simulink model "LCK_old"  (R2018b)
settings: Solver=FixedStepDiscrete  StartTime=0.0  StopTime=inf  FixedStep=0.005  RelTol=1e-3
PostLoadFcn:
  | if any(exist('dsrtsu_mdlpostloadfcn', 'file') ~= 0), dsrtsu_mdlpostloadfcn('Execute', bdroot); end
values from neighbouring files (symbols this model uses):
  C_DEG2RAD = 0.0175    [LCK_Macro.sldd]
  C_KPH2MPS = 0.2778    [LCK_Macro.sldd]
  C_NEARZERO = 0.0001    [LCK_Macro.sldd]
  C_ONE = 1.0    [LCK_Macro.sldd]
  C_RAD2DEG = 57.2958    [LCK_Macro.sldd]
  C_ZERO = 0.0    [LCK_Macro.sldd]
  k_accel_pedal_pos_per_speed_x : value not decoded    [LCK_LogicPara.sldd]
  k_accel_pedal_pos_per_speed_z : value not decoded    [LCK_LogicPara.sldd]
  k_brake_suprress_hold = 1000.0    [LCK_LogicPara.sldd]
  k_driver_appl_torque_filt = 50.0    [LCK_LogicPara.sldd]
  k_driver_suppression_hold_time = 3000.0    [LCK_LogicPara.sldd]
  k_hands_on_wheel_hold_msec = 500.0    [LCK_LogicPara.sldd]
  k_hands_on_wheel_torque_hi = 0.2    [LCK_LogicPara.sldd]
  k_hands_on_wheel_torque_lo = 0.15    [LCK_LogicPara.sldd]
  k_handsoff_delay_cycles = 50.0    [LCK_LogicPara.sldd]
  k_handsoff_torq_Lo_CR = 0.3    [LCK_LogicPara.sldd]
  k_handson_delay_cycles = 5.0    [LCK_LogicPara.sldd]
  k_HighAccel_suppress_hold = 3000.0    [LCK_LogicPara.sldd]
  k_HLR_suprress_hold = 3000.0    [LCK_LogicPara.sldd]
  k_hs_StrAng_CR_threshold_z : value not decoded    [LCK_LogicPara.sldd]
  k_LC_Exit_Switch = 0.0    [LCK_LogicPara.sldd]
  k_LCG_Configured = 1.0    [LCK_LogicPara.sldd]
  k_LCK_A0_Rdy2Act_UseConst = 0.0    [LCK_LogicPara.sldd]
  k_LCK_A0Fac_ActSta : value not decoded    [LCK_CtrlPara.sldd]
  k_LCK_A0Fac_DrvStm : value not decoded    [LCK_CtrlPara.sldd]
  k_LCK_A0Shift_LftCurv : value not decoded    [LCK_CtrlPara.sldd]
  k_LCK_A0Shift_RgtCurv : value not decoded    [LCK_CtrlPara.sldd]
  k_LCK_A0Shift_StraLan = 0.0    [LCK_CtrlPara.sldd]
  k_LCK_A0ShiftFac_Dy_LftCurv : value not decoded    [LCK_CtrlPara.sldd]
  k_LCK_A0ShiftFac_Dy_RgtCurv : value not decoded    [LCK_CtrlPara.sldd]
  k_LCK_A0ShiftFac_Vspd : value not decoded    [LCK_CtrlPara.sldd]
  k_LCK_accel_inhibit_thold = 35.0    [LCK_LogicPara.sldd]
  k_LCK_Active2Ready_Mask = 255.0    [LCK_LogicPara.sldd]
  k_LCK_CvatRateBks : value not decoded    [LCK_CtrlPara.sldd]
  k_LCK_CvatrBks : value not decoded    [LCK_CtrlPara.sldd]
  k_LCK_DFac_Dy : value not decoded    [LCK_CtrlPara.sldd]
  k_LCK_DFac_Dy_Curv : value not decoded    [LCK_CtrlPara.sldd]
  k_LCK_DFac_HaCurCen : value not decoded    [LCK_CtrlPara.sldd]
  k_LCK_DFac_HaCurSid : value not decoded    [LCK_CtrlPara.sldd]
  k_LCK_DFac_HadCurCen : value not decoded    [LCK_CtrlPara.sldd]
  k_LCK_DFac_HadCurSid : value not decoded    [LCK_CtrlPara.sldd]
  k_LCK_DFac_HadStrCen : value not decoded    [LCK_CtrlPara.sldd]
  k_LCK_DFac_HadStrSid : value not decoded    [LCK_CtrlPara.sldd]
  k_LCK_DFac_HaStrCen : value not decoded    [LCK_CtrlPara.sldd]
  k_LCK_DFac_HaStrSid : value not decoded    [LCK_CtrlPara.sldd]
  k_LCK_DFac_Rad : value not decoded    [LCK_CtrlPara.sldd]
  k_LCK_DFac_SA_CurCen : value not decoded    [LCK_CtrlPara.sldd]
  k_LCK_DFac_SA_CurSid : value not decoded    [LCK_CtrlPara.sldd]
  k_LCK_DFac_SA_StrCen : value not decoded    [LCK_CtrlPara.sldd]
  k_LCK_DFac_SA_StrSid : value not decoded    [LCK_CtrlPara.sldd]
  k_LCK_DFac_SS_CurCen : value not decoded    [LCK_CtrlPara.sldd]
  k_LCK_DFac_SS_CurSid : value not decoded    [LCK_CtrlPara.sldd]
  k_LCK_DFac_SS_StrCen : value not decoded    [LCK_CtrlPara.sldd]
  k_LCK_DFac_SS_StrSid : value not decoded    [LCK_CtrlPara.sldd]
  k_LCK_DFac_Vspd : value not decoded    [LCK_CtrlPara.sldd]
  k_LCK_DlyTm_DrvStim = 0.2    [LCK_CtrlPara.sldd]
  k_LCK_DTermMax = 2.0    [LCK_CtrlPara.sldd]
  k_LCK_DyBks_Curv : value not decoded    [LCK_CtrlPara.sldd]
  k_LCK_Enable_POOnly = 1.0    [LCK_LogicPara.sldd]
  k_LCK_Entry_DistBuffer = 0.1    [LCK_LogicPara.sldd]
  k_LCK_Fac_Vspd2RngThr_FalRec = 0.23    [LCK_CtrlPara.sldd]
  k_LCK_Ffw_CvatSwh = 0.0    [LCK_CtrlPara.sldd]
  k_LCK_Ffw_DyBks : value not decoded    [LCK_CtrlPara.sldd]
  k_LCK_Ffw_TimCon_CmdFlt = 0.0    [LCK_CtrlPara.sldd]
  k_LCK_FfwDeltaFac_Rad_Lft : value not decoded    [LCK_CtrlPara.sldd]
  k_LCK_FfwDeltaFac_Rad_Rgt : value not decoded    [LCK_CtrlPara.sldd]
  k_LCK_FfwDeltaFac_Vspd : value not decoded    [LCK_CtrlPara.sldd]
  k_LCK_FfwFac_CvatRate_Lft : value not decoded    [LCK_CtrlPara.sldd]
  k_LCK_FfwFac_CvatRate_Rgt : value not decoded    [LCK_CtrlPara.sldd]
  k_LCK_FfwFac_Dy : value not decoded    [LCK_CtrlPara.sldd]
  k_LCK_FfwFac_Rad_Lft : value not decoded    [LCK_CtrlPara.sldd]
  k_LCK_FfwFac_Rad_Rgt : value not decoded    [LCK_CtrlPara.sldd]
  k_LCK_FfwFac_Vspd : value not decoded    [LCK_CtrlPara.sldd]
  k_LCK_FfwTorq_Cvat : value not decoded    [LCK_CtrlPara.sldd]
  k_LCK_HAFac_ActSta : value not decoded    [LCK_CtrlPara.sldd]
  k_LCK_HAFac_DrvStm : value not decoded    [LCK_CtrlPara.sldd]
  k_LCK_HaloTime = 2000.0    [LCK_LogicPara.sldd]
  k_LCK_HaloTime_Switch = 0.0    [LCK_LogicPara.sldd]
  k_LCK_HARFac_ActSta : value not decoded    [LCK_CtrlPara.sldd]
  k_LCK_HARFac_DrvStm : value not decoded    [LCK_CtrlPara.sldd]
  k_LCK_Hed_DyBks : value not decoded    [LCK_CtrlPara.sldd]
  k_LCK_HedAngDiffX : value not decoded    [LCK_CtrlPara.sldd]
  k_LCK_HedAngRateDiffX : value not decoded    [LCK_CtrlPara.sldd]
  k_LCK_HndsOnWhel_DlyTm_Idl2Rdy = 0.0    [LCK_LogicPara.sldd]
  k_LCK_host_veh_width = 1.86    [LCK_LogicPara.sldd]
  k_LCK_Idle2Ready_Mask = 239.0    [LCK_LogicPara.sldd]
  k_LCK_Junc_SusTime = 1.0    [LCK_LogicPara.sldd]
  k_LCK_KpKdDecSlopeLmt = 10.0    [LCK_CtrlPara.sldd]
  k_LCK_KpKdIncSlopeLmt = 5.0    [LCK_CtrlPara.sldd]
  k_LCK_Lat_Ctrl_DFac_Lft = 1.0    [LCK_CtrlPara.sldd]
  k_LCK_Lat_Ctrl_DFac_Rgt = 1.05    [LCK_CtrlPara.sldd]
  k_LCK_Lat_Ctrl_Kd = 0.8    [LCK_CtrlPara.sldd]
  k_LCK_Lat_Ctrl_Ki = 0.5    [LCK_CtrlPara.sldd]
  k_LCK_Lat_Ctrl_Kp = 0.7    [LCK_CtrlPara.sldd]
  k_LCK_Lat_Ctrl_Kp_NearGain = 0.7    [LCK_CtrlPara.sldd]
  k_LCK_Lat_Ctrl_PFac_Lft = 1.0    [LCK_CtrlPara.sldd]
  k_LCK_Lat_Ctrl_PFac_Rgt = 1.05    [LCK_CtrlPara.sldd]
  k_LCK_Lat_Ctrl_TimCon_CmdFlt = 5.0    [LCK_CtrlPara.sldd]
  k_LCK_Lat_DFac_Rad : value not decoded    [LCK_CtrlPara.sldd]
  k_LCK_Lat_DFac_SS_Cur : value not decoded    [LCK_CtrlPara.sldd]
  k_LCK_Lat_DFac_SS_Str : value not decoded    [LCK_CtrlPara.sldd]
  k_LCK_Lat_DFac_Vspd : value not decoded    [LCK_CtrlPara.sldd]
  k_LCK_Lat_DyBks : value not decoded    [LCK_CtrlPara.sldd]
  k_LCK_Lat_IFac_Rad : value not decoded    [LCK_CtrlPara.sldd]
  k_LCK_Lat_IFac_Vspd : value not decoded    [LCK_CtrlPara.sldd]
  k_LCK_Lat_ILmtFac_Dy_CurvLan : value not decoded    [LCK_CtrlPara.sldd]
  k_LCK_Lat_ILmtFac_Dy_StraLan : value not decoded    [LCK_CtrlPara.sldd]
  k_LCK_Lat_ILmtFac_Rad : value not decoded    [LCK_CtrlPara.sldd]
  k_LCK_Lat_ILmtFac_Rad_NearGain = 1.0    [LCK_CtrlPara.sldd]
  k_LCK_Lat_ILmtFac_Vspd_CurvLan : value not decoded    [LCK_CtrlPara.sldd]
  k_LCK_Lat_ILmtFac_Vspd_StraLan : value not decoded    [LCK_CtrlPara.sldd]
  k_LCK_Lat_ITermLmt_Dy = 1.0    [LCK_CtrlPara.sldd]
  k_LCK_Lat_KpKdDecSlopeLmt = 10.0    [LCK_CtrlPara.sldd]
  k_LCK_Lat_KpKdIncSlopeLmt = 10.0    [LCK_CtrlPara.sldd]
  k_LCK_Lat_PFac_Dy_InnLftCur : value not decoded    [LCK_CtrlPara.sldd]
  k_LCK_Lat_PFac_Dy_InnRgtCur : value not decoded    [LCK_CtrlPara.sldd]
  k_LCK_Lat_PFac_Dy_OutLftCur : value not decoded    [LCK_CtrlPara.sldd]
  k_LCK_Lat_PFac_Dy_OutRgtCur : value not decoded    [LCK_CtrlPara.sldd]
  k_LCK_Lat_PFac_Dy_Str : value not decoded    [LCK_CtrlPara.sldd]
  k_LCK_Lat_PFac_Rad : value not decoded    [LCK_CtrlPara.sldd]
  ... (+158 more)
undefined symbols (not defined in the file or in its folder): k_LCK_CurvBks, K_LCK_SPA0A1A2_LMRngCmp_y
libraries: LateralControl_fcns_lib x58, simulink x22
(part 30 of 45)

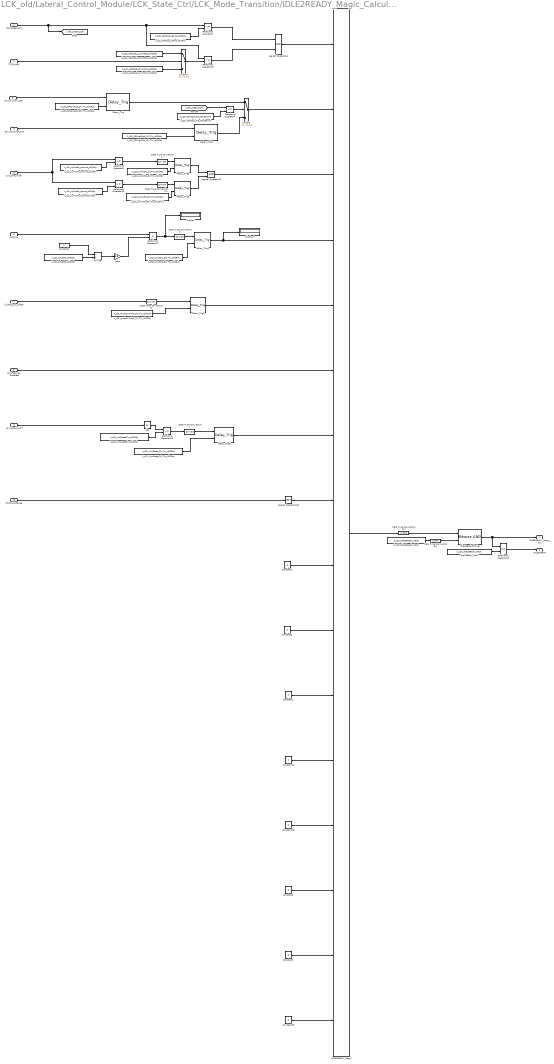
== system LCK_old/Lateral_Control_Module/LCK_State_Ctrl/LCK_Mode_Transition/IDLE2READY_Magic_Calculation ==
  Veh_Speed_kph : Inport
  TJA_Switch : Inport  Port=2
  SP_valid_low_spd : Inport  Port=3
  SP_valid_high_spd : Inport  Port=4
  curr_lane_width : Inport  Port=5
  SPP_A2 : Inport  Port=6
  f_hands_on_wheel : Inport  Port=7
  LCK_Feature_Enabled : Inport  Port=8
  yaw_deg_iso_filt : Inport  Port=9
  Short_LM_Range : Inport  Port=10
  Abs : Abs  Tag={'output',{'type','Float32'},'date',737293.69073196757}  Description=_GWMAB30P4.LCK.000_115_
  Constant1 : Constant  Tag={'output',{'class','ESR_VC/CONST','type','UInt16'},'date',737194.71790592594}  Description=_GWMAB30P2.LCK.000_1070_  Value=0
  Constant11 : Constant  Tag={'output',{'type','Int32'},'date',737237.63745895831}  Description=_GWMAB30P3.LCK.000_18_  Value=0
  Constant15 : Constant  Tag={'output',{'type','Int32'},'date',737504.55055067129}  Description=_GWMAB30P3.LCK.000_21_  Value=0
  Constant16 : Constant  Tag={'output',{'type','Int32'},'date',737237.63745961804}  Description=_GWMAB30P3.LCK.000_22_  Value=0
  Constant2 : Constant  Tag={'output',{'class','ESR_VC/CONST','type','UInt16'},'date',737194.71790592594}  Description=_GWMAB30P2.LCK.000_1070_  Value=0
  Constant3 : Constant  Tag={'output',{'class','ESR_VC/CONST','type','UInt16'},'date',737504.5503860648}  Description=_GWMAB30P2.LCK.000_1079_  Value=0
  Constant4 : Constant  Tag={'output',{'type','Int32'},'date',737296.81489093753}  Description=_GWMAB30P2.LCK.000_1072_
  Constant5 : Constant  Tag={'output',{'class','ESR_VC/CONST','type','UInt16'},'date',737194.71790592594}  Description=_GWMAB30P2.LCK.000_1070_  Value=0
  Constant9 : Constant  Tag={'output',{'class','ESR_VC/CONST','type','UInt16'},'date',737194.71813111112}  Description=_GWMAB30P2.LCK.000_1085_  Value=0
  Data Type Conversion1 : DataTypeConversion  Description=_GWMAB30P4.LCK.000_121_
  Data Type Conversion11 : DataTypeConversion  Description=_GWMAB30P4.LCK.000_122_
  Data Type Conversion12 : DataTypeConversion  Description=_GWMAB30P4.LCK.000_123_  OutDataTypeStr=uint16
  Data Type Conversion21 : DataTypeConversion  Description=_GWMAB30P4.LCK.000_132_
  Data Type Conversion3 : DataTypeConversion  Description=_GWMAB30P4.LCK.000_141_
  Data Type Conversion4 : DataTypeConversion  Description=_GWMAB30P4.LCK.000_146_
  Data Type Conversion93 : DataTypeConversion  OutDataTypeStr=uint16
  Delay_Trig{,1..6} (7 alike) : LateralControl_fcns_lib/Delay_Trig  SystemSampleTime=-1
  Display : Display
  Display1 : Display
  Divide : Product  Inputs=*/
  Gain : Gain  Gain=0.5
  IDLE2READY_Magic : LateralControl_fcns_lib/Bit_To_Integer_16  SystemSampleTime=-1
  "Idle2ReadyBitwise " : simulink/Logic and Bit Operations/Bitwise Operator  logicop=AND  UseBitMask=off  NumInputPorts=2  BitMask=k_LCK_Ready2Idle_Mask  BitMaskRealWorld=Stored Integer
  Idle2Ready_Mask : Constant  Value=k_LCK_Idle2Ready_Mask  SampleTime=-1
  Logical Operator13 : Logic  Tag={'date',737184.60397620371}  Description=_GWMAB30P2.LCK.000_1095_  AllPortsSameDT=off  OutDataTypeStr=boolean
  Logical Operator160 : Logic  Operator=NOT  AllPortsSameDT=off  OutDataTypeStr=boolean
  Logical Operator44 : Logic  Tag={'date',737184.60398003471}  Description=_GWMAB30P2.LCK.000_1126_  AllPortsSameDT=off  OutDataTypeStr=boolean
  Relational Operator10 : RelationalOperator  Tag={'date',737184.60398142366}  Description=_GWMAB30P2.LCK.000_1137_  Operator=<=  OutDataTypeStr=boolean  RndMeth=Nearest
  Relational Operator11 : RelationalOperator  Tag={'date',737184.60398153937}  Description=_GWMAB30P2.LCK.000_1138_  Operator=<  OutDataTypeStr=boolean  RndMeth=Nearest
  Relational Operator15 : RelationalOperator  Tag={'date',737184.60398204857}  Description=_GWMAB30P2.LCK.000_1142_  OutDataTypeStr=boolean  RndMeth=Nearest
  Relational Operator2 : RelationalOperator  Tag={'date',737184.60398265044}  Description=_GWMAB30P2.LCK.000_1147_  Operator=<=  OutDataTypeStr=boolean  RndMeth=Nearest
  Relational Operator29 : RelationalOperator  Tag={'date',737292.69766562502}  Description=_GWMAB30P4.LCK.000_184_  Operator=<=  OutDataTypeStr=boolean  RndMeth=Nearest
  Relational Operator4 : RelationalOperator  Tag={'date',737184.60398497689}  Description=_GWMAB30P2.LCK.000_1166_  Operator=<=  OutDataTypeStr=boolean  RndMeth=Nearest
  Relational Operator9 : RelationalOperator  Tag={'date',737184.6039873379}  Description=_GWMAB30P2.LCK.000_1185_  OutDataTypeStr=boolean  RndMeth=Nearest
  Relational_Operator10 : RelationalOperator  Tag={'date',737184.60398758098}  Description=_GWMAB30P2.LCK.000_1187_  Operator===  OutDataTypeStr=boolean  RndMeth=Nearest
  Switch3 : Switch  Tag={'output',{'inheritscaling',1},'threshold',{'type','Int32','scalar',1},'date',737534.68149979168}  Description=_GWMAB30P2.LCK.000_1193_  Threshold=0.5
  Switch77 : Switch  Tag={'output',{'type','UInt16'},'threshold',{'type','Int32'},'date',737243.53815450228}  Description=_GWMAB30P3.LCK.000_111_  Threshold=0.5
  k_LCK_HndsOnWhel_DlyTm_Idl2Rdy : Constant  Tag={'output',{'name','$P','class','EXTERN_CAL','type','UInt8'},'date',737246.8645407639}  Description=_GWMAB30P2.LCK.000_1235_  Value=k_LCK_HndsOnWhel_DlyTm_Idl2Rdy
  k_LCK_Idle2Ready_Mask : Constant  Value=k_LCK_Idle2Ready_Mask
  k_LCK_LM_ROC_DlyTm_Idl2Rdy : Constant  Tag={'output',{'name','$P','class','EXTERN_CAL','type','UInt8'},'date',737246.86453922454}  Description=_GWMAB30P2.LCK.000_1237_  Value=k_LCK_LM_ROC_DlyTm_Idl2Rdy
  k_LCK_LM_ROC_Idl2Rdy : Constant  Tag={'output',{'name','$P','class','EXTERN_CAL','type','UInt16'},'date',737246.86453881941}  Description=_GWMAB30P2.LCK.000_1239_  Value=k_LCK_LM_ROC_Idl2Rdy
  k_LCK_LnWidth_DlyTm_Idl2Rdy : Constant  Tag={'output',{'name','$P','class','EXTERN_CAL','type','UInt8'},'date',737246.86453662033}  Description=_GWMAB30P2.LCK.000_1243_  Value=k_LCK_LnWidth_DlyTm_Idl2Rdy
  k_LCK_LnWidth_DlyTm_Idl2Rdy1 : Constant  Tag={'output',{'name','$P','class','EXTERN_CAL','type','UInt8'},'date',737246.86453681719}  Description=_GWMAB30P2.LCK.000_1244_  Value=k_LCK_LnWidth_DlyTm_Idl2Rdy
  k_LCK_LnWidth_LowLmt_Idl2Rdy : Constant  Tag={'output',{'name','$P','class','EXTERN_CAL','type','Float32'},'date',737246.86453601858}  Description=_GWMAB30P2.LCK.000_1247_  Value=k_LCK_LnWidth_LowLmt_Idl2Rdy
  k_LCK_LnWidth_UpLmt_Idl2Rdy : Constant  Tag={'output',{'name','$P','class','EXTERN_CAL','type','Float32'},'date',737246.86453563662}  Description=_GWMAB30P2.LCK.000_1249_  Value=k_LCK_LnWidth_UpLmt_Idl2Rdy
  k_LCK_SPHighSpd_DlyTm_Idl2Rdy : Constant  Tag={'output',{'name','$P','class','EXTERN_CAL','type','Float32'},'date',737534.68145640043}  Description=_GWMAB30P2.LCK.000_1228_  Value=k_LCK_SPHighSpd_DlyTm_Idl2Rdy
  k_LCK_SPLowSpd_DlyTm_Idl2Rdy : Constant  Tag={'output',{'name','$P','class','EXTERN_CAL','type','Float32'},'date',737503.62314009259}  Description=_GWMAB30P2.LCK.000_1226_  Value=k_LCK_SPLowSpd_DlyTm_Idl2Rdy
  k_LCK_VehSpd_LowLmtFus_Idl2Rdy : Constant  Tag={'output',{'type','Int32'},'date',737237.63748350693}  Value=k_LCK_VehSpd_LowLmtFus_Idl2Rdy
  k_LCK_VehSpd_LowlmtVis_Idl2Rdy : Constant  Tag={'output',{'name','$P','class','EXTERN_CAL','type','UInt16'},'date',737246.86429228005}  Value=k_LCK_VehSpd_LowlmtVis_Idl2Rdy
  k_LCK_VehSpd_TJA_ICA_Bound : Constant  Tag={'output',{'name','$P','class','EXTERN_CAL','type','UInt16'},'date',737246.86429138889}  Description=_GWMAB30P2.LCK.000_1264_  Value=k_LCK_VehSpd_TJA_ICA_Bound
  k_LCK_VehSpd_Uplmt_Idl2Rdy : Constant  Tag={'output',{'name','$P','class','EXTERN_CAL','type','UInt16'},'date',737246.86429115746}  Description=_GWMAB30P2.LCK.000_1266_  Value=k_LCK_VehSpd_Uplmt_Idl2Rdy
  k_LCK_YawRateThr_Idl2Rdy : Constant  Tag={'output',{'name','$P','class','EXTERN_CAL','type','Float32'},'date',737293.69016506942}  Description=_GWMAB30P4.LCK.000_185_  Value=k_LCK_YawRateThr_Idl2Rdy
  k_LCK_YawRate_DlyTm_Idl2Rdy : Constant  Tag={'output',{'name','$P','class','EXTERN_CAL','type','Float32'},'date',737300.46624641202}  Description=_GWMAB30P4.LCK.000_186_  Value=k_LCK_YawRate_DlyTm_Idl2Rdy
  IDLE2READY_Magic_Out : Outport
  IDLE2READY : Outport  Port=2
  wires:
  Delay_Trig2/1 -> Logical Operator13/1
  Logical Operator160/1 -> IDLE2READY_Magic/8
  Constant1/1 -> IDLE2READY_Magic/9
  k_LCK_VehSpd_LowlmtVis_Idl2Rdy/1 -> Switch77/3
  k_LCK_YawRate_DlyTm_Idl2Rdy/1 -> Delay_Trig6/2
  Delay_Trig3/1 -> Logical Operator13/2
  Data Type Conversion93/1 -> "Idle2ReadyBitwise "/2
  Data Type Conversion12/1 -> "Idle2ReadyBitwise "/1
  Switch3/1 -> IDLE2READY_Magic/2
  Relational Operator29/1 -> Data Type Conversion4/1
  Delay_Trig/1 -> Switch3/1
  Data Type Conversion3/1 -> Delay_Trig4/1
  Idle2Ready_Mask/1 -> Relational_Operator10/2
  Delay_Trig4/1 -> IDLE2READY_Magic/4, Display1/1
  k_LCK_LM_ROC_DlyTm_Idl2Rdy/1 -> Delay_Trig4/2
  Delay_Trig6/1 -> IDLE2READY_Magic/7
  Logical Operator44/1 -> IDLE2READY_Magic/1
  IDLE2READY_Magic/1 -> Data Type Conversion12/1
  Relational Operator2/1 -> Logical Operator44/1
  Veh_Speed_kph/1 -> [veh_speed_kph], Relational Operator2/1, Relational Operator15/1
  Relational Operator10/1 -> Data Type Conversion21/1
  Relational Operator15/1 -> Logical Operator44/2
  Data Type Conversion11/1 -> Delay_Trig5/1
  [veh_speed_kph] -> Relational Operator4/1
  k_LCK_VehSpd_Uplmt_Idl2Rdy/1 -> Relational Operator2/2
  Switch77/1 -> Relational Operator15/2
  Constant16/1 -> IDLE2READY_Magic/13
  Data Type Conversion21/1 -> Delay_Trig3/1
  k_LCK_VehSpd_LowLmtFus_Idl2Rdy/1 -> Switch77/1
  k_LCK_VehSpd_TJA_ICA_Bound/1 -> Relational Operator4/2
  k_LCK_LnWidth_LowLmt_Idl2Rdy/1 -> Relational Operator9/2
  Relational Operator9/1 -> Data Type Conversion1/1
  Data Type Conversion4/1 -> Delay_Trig6/1
  k_LCK_SPLowSpd_DlyTm_Idl2Rdy/1 -> Delay_Trig/2
  k_LCK_SPHighSpd_DlyTm_Idl2Rdy/1 -> Delay_Trig1/2
  Constant3/1 -> IDLE2READY_Magic/14
  Constant2/1 -> IDLE2READY_Magic/11
  Data Type Conversion1/1 -> Delay_Trig2/1
  k_LCK_LnWidth_DlyTm_Idl2Rdy1/1 -> Delay_Trig3/2
  Relational Operator4/1 -> Switch3/2
  Delay_Trig5/1 -> IDLE2READY_Magic/5
  Abs/1 -> Relational Operator29/1
  Constant15/1 -> IDLE2READY_Magic/16
  Relational Operator11/1 -> Display/1, Data Type Conversion3/1
  k_LCK_LnWidth_DlyTm_Idl2Rdy/1 -> Delay_Trig2/2
  Logical Operator13/1 -> IDLE2READY_Magic/3
  Constant11/1 -> IDLE2READY_Magic/12
  k_LCK_LnWidth_UpLmt_Idl2Rdy/1 -> Relational Operator10/2
  Delay_Trig1/1 -> Switch3/3
  k_LCK_YawRateThr_Idl2Rdy/1 -> Relational Operator29/2
  "Idle2ReadyBitwise "/1 -> IDLE2READY_Magic_Out/1, Relational_Operator10/1
  k_LCK_Idle2Ready_Mask/1 -> Data Type Conversion93/1
  Constant9/1 -> IDLE2READY_Magic/15
  k_LCK_HndsOnWhel_DlyTm_Idl2Rdy/1 -> Delay_Trig5/2
  curr_lane_width/1 -> Relational Operator10/1, Relational Operator9/1
  TJA_Switch/1 -> Switch77/2
  Short_LM_Range/1 -> Logical Operator160/1
  f_hands_on_wheel/1 -> Data Type Conversion11/1
  SP_valid_low_spd/1 -> Delay_Trig/1
  Relational_Operator10/1 -> IDLE2READY/1
  SP_valid_high_spd/1 -> Delay_Trig1/1
  LCK_Feature_Enabled/1 -> IDLE2READY_Magic/6
  yaw_deg_iso_filt/1 -> Abs/1
  k_LCK_LM_ROC_Idl2Rdy/1 -> Divide/2
  Constant4/1 -> Divide/1
  Divide/1 -> Gain/1
  Gain/1 -> Relational Operator11/2
  Constant5/1 -> IDLE2READY_Magic/10
  SPP_A2/1 -> Relational Operator11/1
